simulink model "powertrain"  (R2020b)
settings: Solver=FixedStepAuto  StartTime=0.0  StopTime=t(end)  RelTol=1e-3
PreLoadFcn:
  | C_sc = 1;
StartFcn:
  | C_sc = 1;
values from neighbouring files (symbols this model uses):
  D = 0    [model_fc.m]
  Ts = old_data.Ts    [model_fc.m]
undefined symbols (not defined in the file or in its folder): ANFIS, command, DiscIntNeverNeededParam, ECMS, Flight, in, Ion, Lithium, MPC, out, Tmpc, w
libraries: powerlib x25, neural x25, fuzblock x5, electricdrivelib x3, lib_converters x3, simulink x3, re_lib x1
(part 2 of 8)

== system powertrain/Load1/Flight-1 ==
  In1 : Inport
  1-D Lookup Table1 : Lookup_n-D  NumberOfTableDimensions=1  BreakpointsForDimension1=Break1  Table=Scheme1  InternalRulePriority=Speed  RndMeth=Simplest  InputSameDT=on
  Out1 : Outport
  wires:
  1-D Lookup Table1/1 -> Out1/1
  In1/1 -> 1-D Lookup Table1/1

== system powertrain/Load1/Flight-2 ==
  In1 : Inport
  1-D Lookup Table1 : Lookup_n-D  NumberOfTableDimensions=1  BreakpointsForDimension1=Break2  Table=Scheme2  InternalRulePriority=Speed  RndMeth=Simplest  InputSameDT=on
  Out1 : Outport
  wires:
  1-D Lookup Table1/1 -> Out1/1
  In1/1 -> 1-D Lookup Table1/1

== system powertrain/Load1/Flight-3 ==
  In1 : Inport
  1-D Lookup Table1 : Lookup_n-D  NumberOfTableDimensions=1  BreakpointsForDimension1=Break3  Table=Scheme3  InternalRulePriority=Speed  RndMeth=Simplest  InputSameDT=on
  Out1 : Outport
  wires:
  In1/1 -> 1-D Lookup Table1/1
  1-D Lookup Table1/1 -> Out1/1

== system powertrain/Load1/Flight-noise ==
  In1 : Inport
  1-D Lookup Table1 : Lookup_n-D  NumberOfTableDimensions=1  BreakpointsForDimension1=Break4  Table=Scheme4  InternalRulePriority=Speed  RndMeth=Simplest  InputSameDT=on
  Out1 : Outport
  wires:
  In1/1 -> 1-D Lookup Table1/1
  1-D Lookup Table1/1 -> Out1/1

== system powertrain/Load1/Flight-real ==
  In1 : Inport
  1-D Lookup Table1 : Lookup_n-D  NumberOfTableDimensions=1  BreakpointsForDimension1=Break5  Table=Scheme5  InternalRulePriority=Speed  RndMeth=Simplest  InputSameDT=on
  Out1 : Outport
  wires:
  1-D Lookup Table1/1 -> Out1/1
  In1/1 -> 1-D Lookup Table1/1

== system powertrain/Load1/Step ==
  In1 : Inport
  Step : Step  Time=StepTime  Before=InitVal  After=EndVal
  Out1 : Outport
  wires:
  Step/1 -> Out1/1

== system powertrain/Subsystem/Constant ==
  Constant : Constant  Value=irradiance_const
  Out1 : Outport
  wires:
  Constant/1 -> Out1/1

== system powertrain/Subsystem/Model1 ==
  In1 : Inport
  1-D Lookup Table1 : Lookup_n-D  NumberOfTableDimensions=1  BreakpointsForDimension1=break1  Table=irradiance1  InternalRulePriority=Speed  RndMeth=Simplest  InputSameDT=on
  Out1 : Outport
  wires:
  1-D Lookup Table1/1 -> Out1/1
  In1/1 -> 1-D Lookup Table1/1

== system powertrain/Subsystem/Step ==
  Step : Step  Time=break_step  Before=irradiance_step_init  After=irradiance_step_end  SampleTime=0
  Out1 : Outport
  wires:
  Step/1 -> Out1/1

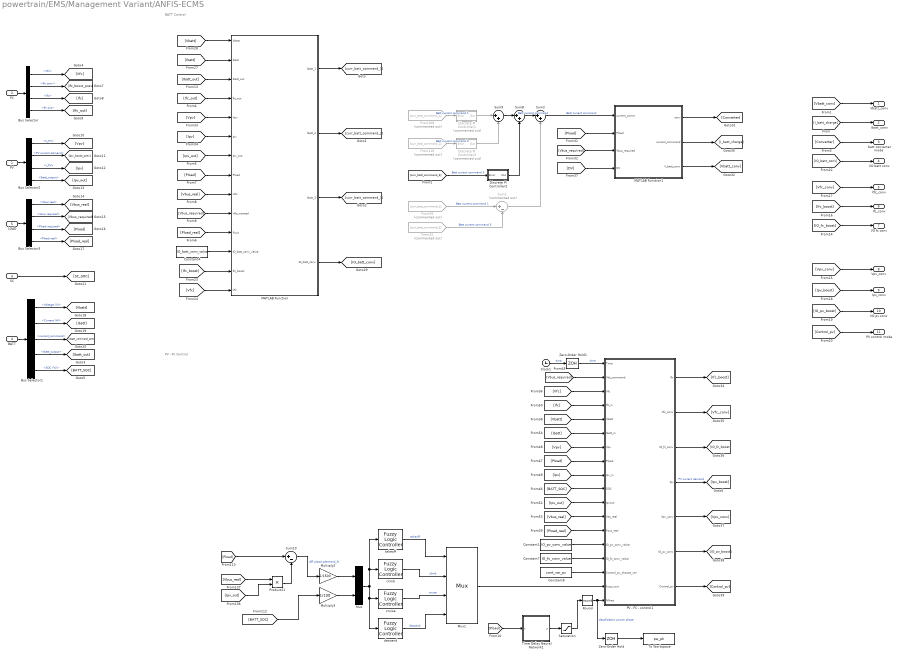
== system powertrain/EMS/Management Variant/ANFIS-ECMS ==
  note: BATT Control
  note: PV - FC Control
  PV : Inport
  FC : Inport  Port=2
  SC : Inport  Port=3
  BATT : Inport  Port=4
  LOAD : Inport  Port=5
  Bus Selector : BusSelector  OutputSignals=Vfc,Ifc conv,Ifc,Ifc out
  Bus Selector1 : BusSelector  OutputSignals=Voltage (V),Current (A),current_command,Ibatt_output,SOC (%)
  Bus Selector2 : BusSelector  OutputSignals=V_PV,PV current demand,I_PV,Ibatt_output
  Bus Selector3 : BusSelector  OutputSignals=Vbus real,Vbus required,Pload required,Pload real
  Clock1 : Clock
  Constant1 : Constant  Value=IO_pv_conv_value
  Constant4 : Constant  Value=IO_batt_conv_value
  Constant7 : Constant  Value=IO_fc_conv_value
  Constant8 : Constant  Value=cont_var_pv
  Discrete PI Controller1 : Subsystem  Commented=on  DialogController=POWERSYS.PowerSysDialog  mask(Discrete PI Controller){Kp=1, Ki=10, Par_Limits=[100 -100], Init=0, Ts=1e-4}
      mask prompts: Kp "Proportional gain (Kp):"; Ki "Integral gain (Ki):"; Par_Limits "Output limits: [ Upper   Lower ]"; Init "Output initial value:"; Ts "Sample time:"
      mask help: This block implements a discrete PI controller.
      mask init:
      | UpperLimit=Par_Limits(1);
      | LowerLimit=Par_Limits(2);
      | power_initmask();
      mask Help: This block is part of a subset of blocks in the Extras library that does not have documentation associated with it, other than the block mask description.
      mask Display: disp('PI');
  Discrete PI Controller2 : Subsystem  DialogController=POWERSYS.PowerSysDialog  mask(Discrete PI Controller){Kp=10, Ki=100, Par_Limits=[30 -4], Init=0, Ts=Ts}
      mask prompts: Kp "Proportional gain (Kp):"; Ki "Integral gain (Ki):"; Par_Limits "Output limits: [ Upper   Lower ]"; Init "Output initial value:"; Ts "Sample time:"
      mask help: This block implements a discrete PI controller.
      mask init:
      | UpperLimit=Par_Limits(1);
      | LowerLimit=Par_Limits(2);
      | power_initmask();
      mask Help: This block is part of a subset of blocks in the Extras library that does not have documentation associated with it, other than the block mask description.
      mask Display: disp('PI');
  Discrete PI Controller3 : Subsystem  Commented=on  DialogController=POWERSYS.PowerSysDialog  mask(Discrete PI Controller){Kp=10, Ki=1, Par_Limits=[100 -100], Init=0, Ts=1e-4}
      mask prompts: Kp "Proportional gain (Kp):"; Ki "Integral gain (Ki):"; Par_Limits "Output limits: [ Upper   Lower ]"; Init "Output initial value:"; Ts "Sample time:"
      mask help: This block implements a discrete PI controller.
      mask init:
      | UpperLimit=Par_Limits(1);
      | LowerLimit=Par_Limits(2);
      | power_initmask();
      mask Help: This block is part of a subset of blocks in the Extras library that does not have documentation associated with it, other than the block mask description.
      mask Display: disp('PI');
  From108 : From  Commented=on  GotoTag=curr_batt_command_1
  From110 : From  Commented=on  GotoTag=curr_batt_command_2
  From25 : From  Commented=on  GotoTag=curr_batt_command_3
  From26 : From  Commented=on  GotoTag=curr_batt_command_1
  MATLAB Function : MATLAB Function  TreatAsAtomicUnit=on
  MATLAB Function1 : MATLAB Function  TreatAsAtomicUnit=on
  Multiply2 : Gain  Gain=1/1500
  Multiply3 : Gain  Gain=1/100
  Mux : Mux  Inputs=2
  Mux1 : Mux
      settings: DisplayOption=signals
  PV - FC - control1 : MATLAB Function  TreatAsAtomicUnit=on
  Product21 : Product
  Round : Rounding  Operator=round
  Saturation : Saturate  UpperLimit=4  LowerLimit=1
  Sum1 : Sum  Commented=on  Inputs=|+-
  Sum10 : Sum  Inputs=|+-
  Sum2 : Sum  Inputs=|++
  Sum8 : Sum  Inputs=|++
  Sum9 : Sum  Inputs=|++
  Time Delay Neural Network1 : Subsystem  mask{pi_input_1_delayed_1=0, pi_input_1_delayed_2=0, pi_input_1_delayed_3=0, pi_input_1_delayed_4=0, pi_input_1_delayed_5=0, pi_input_1_delayed_6=0, pi_input_1_delayed_7=0, pi_input_1_delayed_8=0, pi_input_1_delayed_9=0, pi_input_1_delayed_10=0, pi_input_1_delayed_11=0, pi_input_1_delayed_12=0, pi_input_1_delayed_13=0, pi_input_1_delayed_14=0, pi_input_1_delayed_15=0, pi_input_1_delayed_16=0, pi_input_1_delayed_17=0, pi_input_1_delayed_18=0, pi_input_1_delayed_19=0, pi_input_1_delayed_20=0}
      mask prompts: pi_input_1_delayed_1 "Preprocessed initial input 1 state at timestep 0."; pi_input_1_delayed_2 "Preprocessed initial input 1 state at timestep -1."; pi_input_1_delayed_3 "Preprocessed initial input 1 state at timestep -2."; pi_input_1_delayed_4 "Preprocessed initial input 1 state at timestep -3."; pi_input_1_delayed_5 "Preprocessed initial input 1 state at timestep -4."; pi_input_1_delayed_6 "Preprocessed initial input 1 state at timestep -5."; pi_input_1_delayed_7 "Preprocessed initial input 1 state at timestep -6."; pi_input_1_delayed_8 "Preprocessed initial input 1 state at timestep -7."; pi_input_1_delayed_9 "Preprocessed initial input 1 state at timestep -8."; pi_input_1_delayed_10 "Preprocessed initial input 1 state at timestep -9."; pi_input_1_delayed_11 "Preprocessed initial input 1 state at timestep -10."; pi_input_1_delayed_12 "Preprocessed initial input 1 state at timestep -11."; pi_input_1_delayed_13 "Preprocessed initial input 1 state at timestep -12."; pi_input_1_delayed_14 "Preprocessed initial input 1 state at timestep -13."; pi_input_1_delayed_15 "Preprocessed initial input 1 state at timestep -14."; pi_input_1_delayed_16 "Preprocessed initial input 1 state at timestep -15."; pi_input_1_delayed_17 "Preprocessed initial input 1 state at timestep -16."; pi_input_1_delayed_18 "Preprocessed initial input 1 state at timestep -17."; pi_input_1_delayed_19 "Preprocessed initial input 1 state at timestep -18."; pi_input_1_delayed_20 "Preprocessed initial input 1 state at timestep -19."
      mask help: Time Delay Neural Network
      mask Display: e = 0.06;c1 = [120 150 230]/255;c2 = ([120 150 230]+0)/383;c3 = ([120 150 230]+128)/383;patch([0 1 1 0],[0 0 1 1],c1);patch([0 1 1 1-e 1-e 0+e],[0 0 1 1-e 0+e 0+e],c2);patch([0 0 1 1-e 0+e 0+e],[0 1 1 1-e 1-e 0+e],c3);plot([0 1 1 0 0],[0 0 1 1 0]);fprintf('NNET');port_label('input',1,' x');port_label('output',1,'y ');
  To Workspace : ToWorkspace  VariableName=pw_ph  SaveFormat=Timeseries  SampleTime=-1
  Zero-Order Hold : ZeroOrderHold  SampleTime=Ts
  Zero-Order Hold1 : ZeroOrderHold  SampleTime=Ts
  climb : fuzblock/Fuzzy Logic  Controller  FIS='B80_ECMS_climb.fis'  OutputSampleNumber=10  DataType=double  FuzzifiedInputs=off  RuleFiringStrengths=off  RuleOutputs=off  AggregatedOutputs=off  SimulateUsing=Code generation  OutOfRangeInputValueMessage=warning  NoRuleFiredMessage=warning  EmptyOutputFuzzySetMessage=warning
  cruise : fuzblock/Fuzzy Logic  Controller  FIS='B80_ECMS_cruise.fis'  OutputSampleNumber=10  DataType=double  FuzzifiedInputs=off  RuleFiringStrengths=off  RuleOutputs=off  AggregatedOutputs=off  SimulateUsing=Code generation  OutOfRangeInputValueMessage=warning  NoRuleFiredMessage=warning  EmptyOutputFuzzySetMessage=warning
  descend : fuzblock/Fuzzy Logic  Controller  FIS='B80_ECMS_descend.fis'  OutputSampleNumber=10  DataType=double  FuzzifiedInputs=off  RuleFiringStrengths=off  RuleOutputs=off  AggregatedOutputs=off  SimulateUsing=Code generation  OutOfRangeInputValueMessage=warning  NoRuleFiredMessage=warning  EmptyOutputFuzzySetMessage=warning
  takeoff : fuzblock/Fuzzy Logic  Controller  FIS='B80_ECMS_takeoff.fis'  OutputSampleNumber=10  DataType=double  FuzzifiedInputs=off  RuleFiringStrengths=off  RuleOutputs=off  AggregatedOutputs=off  SimulateUsing=Code generation  OutOfRangeInputValueMessage=warning  NoRuleFiredMessage=warning  EmptyOutputFuzzySetMessage=warning
  Vbatt_conv : Outport
  Ibatt_conv : Outport  Port=2
  batt converter mode : Outport  Port=3
  I/O batt conv : Outport  Port=4
  Vfc_conv : Outport  Port=5
  Ifc_conv : Outport  Port=6
  I/O fc conv : Outport  Port=7
  Vpv_conv : Outport  Port=8
  Ipv_conv : Outport  Port=9
  I/O pv conv : Outport  Port=10
  PV control mode : Outport  Port=11
  wires:
  [DV] -> MATLAB Function1/4(DV)
  Discrete PI Controller1/1(Out) -> Sum9/1
  [I_batt_charge] -> Ibatt_conv/1
  MATLAB Function1/1(conv) -> [Converter]
  [Converter] -> batt converter mode/1
  Sum9/1 -> Sum8/1
  Bus Selector1/1 -> [Vbatt]  "<Voltage (V)>"
  [Vbus_real] -> MATLAB Function/9(Vdc)
  [Vpv] -> MATLAB Function/5(Vpv)
  Bus Selector/1 -> [Vfc]  "<Vfc>"
  Sum2/1 -> MATLAB Function1/1(current_comm)  "Batt current command"
  [Vfc_conv] -> Vfc_conv/1
  BATT/1 -> Bus Selector1/1
  From25/1 -> Sum1/2  "Batt current command 3"
  MATLAB Function/3(Ibatt_3) -> [curr_batt_command_3]
  [Vfc] -> MATLAB Function/14(Vfc)
  Bus Selector2/3 -> [Ipv]  "<I_PV>"
  [IO_pv_boost] -> I/O pv conv/1
  From108/1 -> Discrete PI Controller1/1(Error)  "Batt current command 1"
  [Ibatt] -> MATLAB Function/2(Ibatt)
  [IO_fc_boost] -> I/O fc conv/1
  MATLAB Function/2(Ibatt_2) -> [curr_batt_command_2]
  Constant4/1 -> MATLAB Function/12(IO_batt_conv_value)
  MATLAB Function/1(Ibatt_1) -> [curr_batt_command_1]
  [Pload] -> MATLAB Function1/2(Pload)
  Bus Selector2/1 -> [Vpv]  "<V_PV>"
  [Ipv] -> MATLAB Function/6(Ipv)
  SC/1 -> [SC_SOC]
  [Ibatt_out] -> MATLAB Function/3(Ibatt_out)
  MATLAB Function1/2(current_command) -> [I_batt_charge]
  [Pload_real] -> MATLAB Function/11(Pout)
  From26/1 -> Sum1/1  "Batt current command 1"
  Bus Selector/4 -> [Ifc_out]  "<Ifc out>"
  FC/1 -> Bus Selector/1
  Bus Selector2/2 -> [Ipv_boost_prev]  "<PV current demand>"
  Bus Selector3/1 -> [Vbus_real]  "<Vbus real>"
  Bus Selector3/2 -> [Vbus_required]  "<Vbus required>"
  [Ipv_boost] -> Ipv_conv/1
  Bus Selector1/4 -> [Ibatt_out]  "<Ibatt_output>"
  Bus Selector1/5 -> [BATT_SOC]  "<SOC (%)>"
  Discrete PI Controller2/1(Out) -> Sum8/2
  [Vbatt] -> MATLAB Function/1(Vbatt)
  Discrete PI Controller3/1(Out) -> Sum9/2
  Bus Selector3/4 -> [Pload_real]  "<Pload real>"
  Bus Selector/2 -> [Ifc_boost_prev]  "<Ifc conv>"
  [Ifc_boost] -> MATLAB Function/13(Ifc_boost)
  MATLAB Function1/3(V_batt_conv) -> [Vbatt_conv]
  Bus Selector1/2 -> [Ibatt]  "<Current (A)>"
  [Vpv_conv] -> Vpv_conv/1
  [Ifc_out] -> MATLAB Function/4(Ifc_out)
  Bus Selector1/3 -> [Ibatt_command_pre]  "<current_command>"
  [Vbus_required] -> MATLAB Function1/3(Vbus_required)
  From110/1 -> Discrete PI Controller3/1(Error)  "Batt current command 3"
  [curr_batt_command_3] -> Discrete PI Controller2/1(Error)  "Batt current command 3"
  PV/1 -> Bus Selector2/1
  [Vbus_required] -> MATLAB Function/10(Vdc_wanted)
  Bus Selector2/4 -> [Ipv_out]  "<Ibatt_output>"
  Bus Selector3/3 -> [Pload]  "<Pload required>"
  [IO_batt_conv] -> I/O batt conv/1
  Bus Selector/3 -> [Ifc]  "<Ifc>"
  [Ipv_out] -> MATLAB Function/7(Ipv_out)
  [Control_pv] -> PV control mode/1
  LOAD/1 -> Bus Selector3/1
  Sum8/1 -> Sum2/1  "Batt current command"
  [Pload] -> MATLAB Function/8(Pload)
  [Vbatt_conv] -> Vbatt_conv/1
  MATLAB Function/4(IO_batt_conv) -> [IO_batt_conv]
  Sum1/1 -> Sum2/2
  [Vbus_real] -> Product21/1
  takeoff/1 -> Mux1/1  "takeoff"
  [BATT_SOC] -> Multiply3/1
  Multiply2/1 -> Mux/1
  [Pload] -> Sum10/1
  Product21/1 -> Sum10/2
  Mux/1 -> takeoff/1, climb/1, descend/1, cruise/1
  Sum10/1 -> Multiply2/1  "diff pload pdemand_fc"
  [Ipv_out] -> Product21/2
  Multiply3/1 -> Mux/2
  Mux1/1 -> PV - FC - control1/17(fuzzy_out)
  PV - FC - control1/1(Ifc) -> [Ifc_boost]
  Zero-Order Hold1/1 -> PV - FC - control1/1(Time)  "time"
  [Pload] -> PV - FC - control1/8(Pload)
  Constant7/1 -> PV - FC - control1/15(IO_fc_conv_value)
  [BATT_SOC] -> PV - FC - control1/10(SOC)
  [Vbatt] -> PV - FC - control1/5(Vbatt)
  [Ibatt] -> PV - FC - control1/6(Ibatt_in)
  PV - FC - control1/5(Vpv_conv) -> [Vpv_conv]
  PV - FC - control1/2(Vfc_conv) -> [Vfc_conv]
  [Vfc] -> PV - FC - control1/3(Vfc)
  PV - FC - control1/4(Ipv) -> [Ipv_boost]  "PV current demand"
  [Ifc] -> PV - FC - control1/4(Ifc_in)
  Constant8/1 -> PV - FC - control1/16(Control_pv_choose_var)
  [Ipv] -> PV - FC - control1/9(Ipv_in)
  PV - FC - control1/6(IO_pv_conv) -> [IO_pv_boost]
  [Pload_real] -> PV - FC - control1/13(Pout_real)
  PV - FC - control1/7(Control_pv) -> [Control_pv]
  [Vbus_real] -> PV - FC - control1/12(Vdc_real)
  [Vpv] -> PV - FC - control1/7(Vpv)
  Constant1/1 -> PV - FC - control1/14(IO_pv_conv_value)
  [Ipv_out] -> PV - FC - control1/11(Ipvout)
  Clock1/1 -> Zero-Order Hold1/1  "time"
  [Vbus_required] -> PV - FC - control1/2(Vdc_command)
  PV - FC - control1/3(IO_fc_conv) -> [IO_fc_boost]
  climb/1 -> Mux1/2  "climb"
  cruise/1 -> Mux1/3  "cruise"
  descend/1 -> Mux1/4  "descend"
  Time Delay Neural Network1/1(y) -> Saturation/1
  [Pload] -> Time Delay Neural Network1/1(x)
  Saturation/1 -> Round/1
  Round/1 -> Zero-Order Hold/1, PV - FC - control1/18(NNres)  "classficiation power phase"
  [Ifc_boost] -> Ifc_conv/1
  Zero-Order Hold/1 -> To Workspace/1

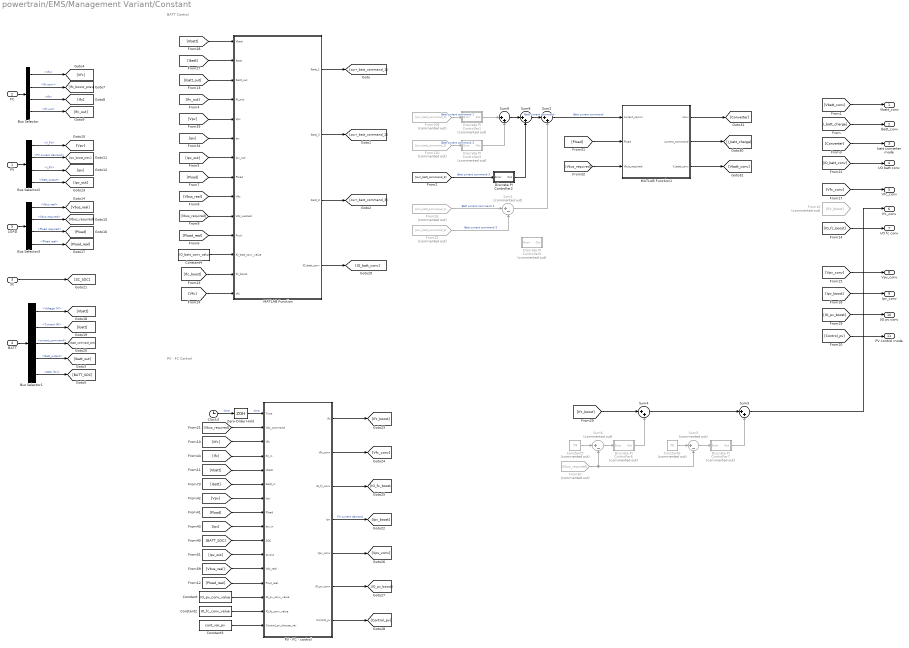
== system powertrain/EMS/Management Variant/Constant ==
  note: BATT Control
  note: PV - FC Control
  PV : Inport
  FC : Inport  Port=2
  SC : Inport  Port=3
  BATT : Inport  Port=4
  LOAD : Inport  Port=5
  Bus Selector : BusSelector  OutputSignals=Vfc,Ifc conv,Ifc,Ifc out
  Bus Selector1 : BusSelector  OutputSignals=Voltage (V),Current (A),current_command,Ibatt_output,SOC (%)
  Bus Selector2 : BusSelector  OutputSignals=V_PV,PV current demand,I_PV,Ibatt_output
  Bus Selector3 : BusSelector  OutputSignals=Vbus real,Vbus required,Pload required,Pload real
  Clock3 : Clock
  Constant : Constant  Value=IO_pv_conv_value
  Constant2 : Constant  Value=IO_fc_conv_value
  Constant3 : Constant  Value=cont_var_pv
  Constant4 : Constant  Value=IO_batt_conv_value
  Constant5 : Constant  Commented=on  Value=74
  Constant6 : Constant  Commented=on  Value=70
  Discrete PI Controller1 : Subsystem  Commented=on  DialogController=POWERSYS.PowerSysDialog  mask(Discrete PI Controller){Kp=1, Ki=10, Par_Limits=[100 -100], Init=0, Ts=1e-4}
      mask prompts: Kp "Proportional gain (Kp):"; Ki "Integral gain (Ki):"; Par_Limits "Output limits: [ Upper   Lower ]"; Init "Output initial value:"; Ts "Sample time:"
      mask help: This block implements a discrete PI controller.
      mask init:
      | UpperLimit=Par_Limits(1);
      | LowerLimit=Par_Limits(2);
      | power_initmask();
      mask Help: This block is part of a subset of blocks in the Extras library that does not have documentation associated with it, other than the block mask description.
      mask Display: disp('PI');
  Discrete PI Controller2 : Subsystem  DialogController=POWERSYS.PowerSysDialog  mask(Discrete PI Controller){Kp=10, Ki=100, Par_Limits=[30 -4], Init=0, Ts=Ts}
      mask prompts: Kp "Proportional gain (Kp):"; Ki "Integral gain (Ki):"; Par_Limits "Output limits: [ Upper   Lower ]"; Init "Output initial value:"; Ts "Sample time:"
      mask help: This block implements a discrete PI controller.
      mask init:
      | UpperLimit=Par_Limits(1);
      | LowerLimit=Par_Limits(2);
      | power_initmask();
      mask Help: This block is part of a subset of blocks in the Extras library that does not have documentation associated with it, other than the block mask description.
      mask Display: disp('PI');
  Discrete PI Controller3 : Subsystem  Commented=on  DialogController=POWERSYS.PowerSysDialog  mask(Discrete PI Controller){Kp=10, Ki=1, Par_Limits=[100 -100], Init=0, Ts=1e-4}
      mask prompts: Kp "Proportional gain (Kp):"; Ki "Integral gain (Ki):"; Par_Limits "Output limits: [ Upper   Lower ]"; Init "Output initial value:"; Ts "Sample time:"
      mask help: This block implements a discrete PI controller.
      mask init:
      | UpperLimit=Par_Limits(1);
      | LowerLimit=Par_Limits(2);
      | power_initmask();
      mask Help: This block is part of a subset of blocks in the Extras library that does not have documentation associated with it, other than the block mask description.
      mask Display: disp('PI');
  Discrete PI Controller5 : Subsystem  Commented=on  DialogController=POWERSYS.PowerSysDialog  mask(Discrete PI Controller){Kp=10, Ki=10, Par_Limits=[50 -20], Init=0, Ts=1e-4}
      mask prompts: Kp "Proportional gain (Kp):"; Ki "Integral gain (Ki):"; Par_Limits "Output limits: [ Upper   Lower ]"; Init "Output initial value:"; Ts "Sample time:"
      mask help: This block implements a discrete PI controller.
      mask init:
      | UpperLimit=Par_Limits(1);
      | LowerLimit=Par_Limits(2);
      | power_initmask();
      mask Help: This block is part of a subset of blocks in the Extras library that does not have documentation associated with it, other than the block mask description.
      mask Display: disp('PI');
  Discrete PI Controller6 : Subsystem  Commented=on  DialogController=POWERSYS.PowerSysDialog  mask(Discrete PI Controller){Kp=10, Ki=10, Par_Limits=[40 0], Init=0, Ts=1e-4}
      mask prompts: Kp "Proportional gain (Kp):"; Ki "Integral gain (Ki):"; Par_Limits "Output limits: [ Upper   Lower ]"; Init "Output initial value:"; Ts "Sample time:"
      mask help: This block implements a discrete PI controller.
      mask init:
      | UpperLimit=Par_Limits(1);
      | LowerLimit=Par_Limits(2);
      | power_initmask();
      mask Help: This block is part of a subset of blocks in the Extras library that does not have documentation associated with it, other than the block mask description.
      mask Display: disp('PI');
  Discrete PI Controller7 : Subsystem  Commented=on  DialogController=POWERSYS.PowerSysDialog  mask(Discrete PI Controller){Kp=10, Ki=10, Par_Limits=[0 -40], Init=0, Ts=1e-4}
      mask prompts: Kp "Proportional gain (Kp):"; Ki "Integral gain (Ki):"; Par_Limits "Output limits: [ Upper   Lower ]"; Init "Output initial value:"; Ts "Sample time:"
      mask help: This block implements a discrete PI controller.
      mask init:
      | UpperLimit=Par_Limits(1);
      | LowerLimit=Par_Limits(2);
      | power_initmask();
      mask Help: This block is part of a subset of blocks in the Extras library that does not have documentation associated with it, other than the block mask description.
      mask Display: disp('PI');
  From108 : From  Commented=on  GotoTag=curr_batt_command_1
  From110 : From  Commented=on  GotoTag=curr_batt_command_2
  From16 : From  Commented=on  GotoTag=Ifc_boost
  From25 : From  Commented=on  GotoTag=curr_batt_command_3
  From26 : From  Commented=on  GotoTag=curr_batt_command_1
  From30 : From  Commented=on  GotoTag=Vbus_required
  MATLAB Function : MATLAB Function  TreatAsAtomicUnit=on
  MATLAB Function1 : MATLAB Function  TreatAsAtomicUnit=on
  PV - FC - control : MATLAB Function  TreatAsAtomicUnit=on
  Sum1 : Sum  Commented=on  Inputs=|+-
  Sum{2..4,8..9} (5 alike) : Sum  Inputs=|++
  Sum5 : Sum  Commented=on  Inputs=|+-
  Sum6 : Sum  Commented=on  Inputs=|+-
  Zero-Order Hold : ZeroOrderHold  SampleTime=1e-4
  Vbatt_conv : Outport
  Ibatt_conv : Outport  Port=2
  batt converter mode : Outport  Port=3
  I/O batt conv : Outport  Port=4
  Vfc_conv : Outport  Port=5
  Ifc_conv : Outport  Port=6
  I/O fc conv : Outport  Port=7
  Vpv_conv : Outport  Port=8
  Ipv_conv : Outport  Port=9
  I/O pv conv : Outport  Port=10
  PV control mode : Outport  Port=11
  wires:
  Constant/1 -> PV - FC - control/14(IO_pv_conv_value)
  MATLAB Function1/1(conv) -> [Converter]
  [Vbatt] -> MATLAB Function/1(Vbatt)
  [Ibatt_out] -> MATLAB Function/3(Ibatt_out)
  Bus Selector1/5 -> [BATT_SOC]  "<SOC (%)>"
  From30/1 -> Sum5/2, Sum6/2
  [Vpv] -> MATLAB Function/5(Vpv)
  Sum6/1 -> Discrete PI Controller6/1(Error)
  Discrete PI Controller7/1(Out) -> Sum3/2
  PV - FC - control/3(IO_fc_conv) -> [IO_fc_boost]
  [Ifc_out] -> MATLAB Function/4(Ifc_out)
  Bus Selector1/3 -> [Ibatt_command_pre]  "<current_command>"
  [IO_fc_boost] -> I/O fc conv/1
  MATLAB Function1/3(V_batt_conv) -> [Vbatt_conv]
  Bus Selector1/2 -> [Ibatt]  "<Current (A)>"
  [Ifc_boost] -> MATLAB Function/13(Ifc_boost)
  [Vbus_required] -> MATLAB Function1/3(Vbus_required)
  Sum2/1 -> MATLAB Function1/1(current_comm)  "Batt current command"
  [Vpv_conv] -> Vpv_conv/1
  Bus Selector1/1 -> [Vbatt]  "<Voltage (V)>"
  [Ibatt] -> PV - FC - control/6(Ibatt_in)
  From26/1 -> Sum1/1  "Batt current command 1"
  Bus Selector1/4 -> [Ibatt_out]  "<Ibatt_output>"
  MATLAB Function1/2(current_command) -> [I_batt_charge]
  [Ipv_boost] -> Ipv_conv/1
  [Pload_real] -> MATLAB Function/11(Pout)
  PV - FC - control/5(Vpv_conv) -> [Vpv_conv]
  Constant6/1 -> Sum5/1
  Sum5/1 -> Discrete PI Controller7/1(Error)
  Constant2/1 -> PV - FC - control/15(IO_fc_conv_value)
  MATLAB Function/2(Ibatt_2) -> [curr_batt_command_2]
  MATLAB Function/1(Ibatt_1) -> [curr_batt_command_1]
  Bus Selector2/1 -> [Vpv]  "<V_PV>"
  [Pload] -> MATLAB Function1/2(Pload)
  Sum4/1 -> Sum3/1
  [Ifc_boost] -> Sum4/1
  From25/1 -> Sum1/2  "Batt current command 3"
  [Ibatt] -> MATLAB Function/2(Ibatt)
  [IO_pv_boost] -> I/O pv conv/1
  [Vfc] -> MATLAB Function/14(Vfc)
  Bus Selector2/3 -> [Ipv]  "<I_PV>"
  Sum1/1 -> Sum2/2
  [Vfc_conv] -> Vfc_conv/1
  [Ipv_out] -> PV - FC - control/11(Ipvout)
  PV - FC - control/7(Control_pv) -> [Control_pv]
  [Vbus_required] -> PV - FC - control/2(Vdc_command)
  [Vbatt_conv] -> Vbatt_conv/1
  [Vbus_real] -> PV - FC - control/12(Vdc_real)
  MATLAB Function/4(IO_batt_conv) -> [IO_batt_conv]
  Constant3/1 -> PV - FC - control/16(Control_pv_choose_var)
  PV - FC - control/1(Ifc) -> [Ifc_boost]
  FC/1 -> Bus Selector/1
  [Ipv] -> PV - FC - control/9(Ipv_in)
  Sum8/1 -> Sum2/1  "Batt current command"
  Zero-Order Hold/1 -> PV - FC - control/1(Time)  "time"
  [Pload] -> MATLAB Function/8(Pload)
  [Vbus_required] -> MATLAB Function/10(Vdc_wanted)
  Clock3/1 -> Zero-Order Hold/1  "time"
  [Pload_real] -> PV - FC - control/13(Pout_real)
  [Vpv] -> PV - FC - control/7(Vpv)
  LOAD/1 -> Bus Selector3/1
  Constant5/1 -> Sum6/1
  [Control_pv] -> PV control mode/1
  Bus Selector/3 -> [Ifc]  "<Ifc>"
  [Ipv_out] -> MATLAB Function/7(Ipv_out)
  From110/1 -> Discrete PI Controller3/1(Error)  "Batt current command 3"
  [IO_batt_conv] -> I/O batt conv/1
  [Vbus_real] -> MATLAB Function/9(Vdc)
  Bus Selector3/3 -> [Pload]  "<Pload required>"
  Bus Selector2/4 -> [Ipv_out]  "<Ibatt_output>"
  PV - FC - control/4(Ipv) -> [Ipv_boost]  "PV current demand"
  [Ifc] -> PV - FC - control/4(Ifc_in)
  Bus Selector3/2 -> [Vbus_required]  "<Vbus required>"
  BATT/1 -> Bus Selector1/1
  Discrete PI Controller6/1(Out) -> Sum4/2
  Bus Selector2/2 -> [Ipv_boost_prev]  "<PV current demand>"
  Bus Selector3/1 -> [Vbus_real]  "<Vbus real>"
  Constant4/1 -> MATLAB Function/12(IO_batt_conv_value)
  PV - FC - control/6(IO_pv_conv) -> [IO_pv_boost]
  SC/1 -> [SC_SOC]
  [Converter] -> batt converter mode/1
  PV - FC - control/2(Vfc_conv) -> [Vfc_conv]
  [I_batt_charge] -> Ibatt_conv/1
  [Vbatt] -> PV - FC - control/5(Vbatt)
  [Vfc] -> PV - FC - control/3(Vfc)
  [curr_batt_command_3] -> Discrete PI Controller2/1(Error)  "Batt current command 3"
  Bus Selector/1 -> [Vfc]  "<Vfc>"
  Bus Selector/4 -> [Ifc_out]  "<Ifc out>"
  PV/1 -> Bus Selector2/1
  [Pload] -> PV - FC - control/8(Pload)
  Bus Selector/2 -> [Ifc_boost_prev]  "<Ifc conv>"
  Sum9/1 -> Sum8/1
  From108/1 -> Discrete PI Controller1/1(Error)  "Batt current command 1"
  Discrete PI Controller2/1(Out) -> Sum8/2
  MATLAB Function/3(Ibatt_3) -> [curr_batt_command_3]
  Sum3/1 -> Ifc_conv/1
  Discrete PI Controller1/1(Out) -> Sum9/1
  Discrete PI Controller3/1(Out) -> Sum9/2
  [BATT_SOC] -> PV - FC - control/10(SOC)
  [Ipv] -> MATLAB Function/6(Ipv)
  Bus Selector3/4 -> [Pload_real]  "<Pload real>"

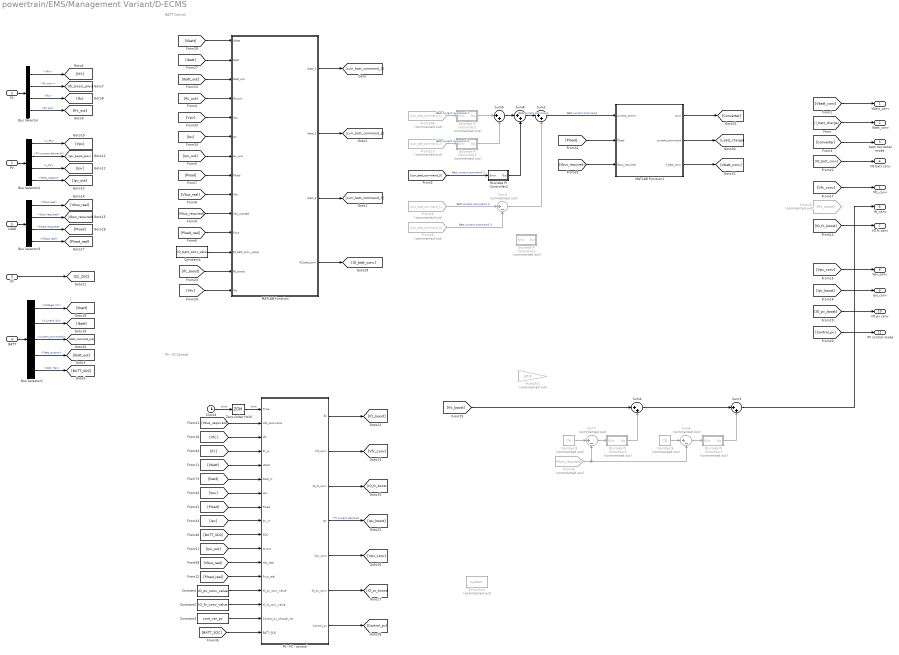
== system powertrain/EMS/Management Variant/D-ECMS ==
  note: PV - FC Control
  note: BATT Control
  PV : Inport
  FC : Inport  Port=2
  SC : Inport  Port=3
  BATT : Inport  Port=4
  LOAD : Inport  Port=5
  Bus Selector : BusSelector  OutputSignals=Vfc,Ifc conv,Ifc,Ifc out
  Bus Selector1 : BusSelector  OutputSignals=Voltage (V),Current (A),current_command,Ibatt_output,SOC (%)
  Bus Selector2 : BusSelector  OutputSignals=V_PV,PV current demand,I_PV,Ibatt_output
  Bus Selector3 : BusSelector  OutputSignals=Vbus real,Vbus required,Pload required,Pload real
  Clock3 : Clock
  Constant : Constant  Value=IO_pv_conv_value
  Constant2 : Constant  Value=IO_fc_conv_value
  Constant3 : Constant  Value=cont_var_pv
  Constant4 : Constant  Value=IO_batt_conv_value
  Constant5 : Constant  Commented=on  Value=74
  Constant6 : Constant  Commented=on  Value=70
  Discrete PI Controller1 : Subsystem  Commented=on  DialogController=POWERSYS.PowerSysDialog  mask(Discrete PI Controller){Kp=1, Ki=10, Par_Limits=[100 -100], Init=0, Ts=1e-4}
      mask prompts: Kp "Proportional gain (Kp):"; Ki "Integral gain (Ki):"; Par_Limits "Output limits: [ Upper   Lower ]"; Init "Output initial value:"; Ts "Sample time:"
      mask help: This block implements a discrete PI controller.
      mask init:
      | UpperLimit=Par_Limits(1);
      | LowerLimit=Par_Limits(2);
      | power_initmask();
      mask Help: This block is part of a subset of blocks in the Extras library that does not have documentation associated with it, other than the block mask description.
      mask Display: disp('PI');
  Discrete PI Controller2 : Subsystem  DialogController=POWERSYS.PowerSysDialog  mask(Discrete PI Controller){Kp=10, Ki=100, Par_Limits=[30 -4], Init=0, Ts=Ts}
      mask prompts: Kp "Proportional gain (Kp):"; Ki "Integral gain (Ki):"; Par_Limits "Output limits: [ Upper   Lower ]"; Init "Output initial value:"; Ts "Sample time:"
      mask help: This block implements a discrete PI controller.
      mask init:
      | UpperLimit=Par_Limits(1);
      | LowerLimit=Par_Limits(2);
      | power_initmask();
      mask Help: This block is part of a subset of blocks in the Extras library that does not have documentation associated with it, other than the block mask description.
      mask Display: disp('PI');
  Discrete PI Controller3 : Subsystem  Commented=on  DialogController=POWERSYS.PowerSysDialog  mask(Discrete PI Controller){Kp=10, Ki=1, Par_Limits=[100 -100], Init=0, Ts=1e-4}
      mask prompts: Kp "Proportional gain (Kp):"; Ki "Integral gain (Ki):"; Par_Limits "Output limits: [ Upper   Lower ]"; Init "Output initial value:"; Ts "Sample time:"
      mask help: This block implements a discrete PI controller.
      mask init:
      | UpperLimit=Par_Limits(1);
      | LowerLimit=Par_Limits(2);
      | power_initmask();
      mask Help: This block is part of a subset of blocks in the Extras library that does not have documentation associated with it, other than the block mask description.
      mask Display: disp('PI');
  Discrete PI Controller5 : Subsystem  Commented=on  DialogController=POWERSYS.PowerSysDialog  mask(Discrete PI Controller){Kp=10, Ki=10, Par_Limits=[50 -20], Init=0, Ts=1e-4}
      mask prompts: Kp "Proportional gain (Kp):"; Ki "Integral gain (Ki):"; Par_Limits "Output limits: [ Upper   Lower ]"; Init "Output initial value:"; Ts "Sample time:"
      mask help: This block implements a discrete PI controller.
      mask init:
      | UpperLimit=Par_Limits(1);
      | LowerLimit=Par_Limits(2);
      | power_initmask();
      mask Help: This block is part of a subset of blocks in the Extras library that does not have documentation associated with it, other than the block mask description.
      mask Display: disp('PI');
  Discrete PI Controller6 : Subsystem  Commented=on  DialogController=POWERSYS.PowerSysDialog  mask(Discrete PI Controller){Kp=10, Ki=10, Par_Limits=[40 0], Init=0, Ts=1e-4}
      mask prompts: Kp "Proportional gain (Kp):"; Ki "Integral gain (Ki):"; Par_Limits "Output limits: [ Upper   Lower ]"; Init "Output initial value:"; Ts "Sample time:"
      mask help: This block implements a discrete PI controller.
      mask init:
      | UpperLimit=Par_Limits(1);
      | LowerLimit=Par_Limits(2);
      | power_initmask();
      mask Help: This block is part of a subset of blocks in the Extras library that does not have documentation associated with it, other than the block mask description.
      mask Display: disp('PI');
  Discrete PI Controller7 : Subsystem  Commented=on  DialogController=POWERSYS.PowerSysDialog  mask(Discrete PI Controller){Kp=10, Ki=10, Par_Limits=[0 -40], Init=0, Ts=1e-4}
      mask prompts: Kp "Proportional gain (Kp):"; Ki "Integral gain (Ki):"; Par_Limits "Output limits: [ Upper   Lower ]"; Init "Output initial value:"; Ts "Sample time:"
      mask help: This block implements a discrete PI controller.
      mask init:
      | UpperLimit=Par_Limits(1);
      | LowerLimit=Par_Limits(2);
      | power_initmask();
      mask Help: This block is part of a subset of blocks in the Extras library that does not have documentation associated with it, other than the block mask description.
      mask Display: disp('PI');
  From108 : From  Commented=on  GotoTag=curr_batt_command_1
  From110 : From  Commented=on  GotoTag=curr_batt_command_2
  From16 : From  Commented=on  GotoTag=Ifc_boost
  From25 : From  Commented=on  GotoTag=curr_batt_command_3
  From26 : From  Commented=on  GotoTag=curr_batt_command_1
  From30 : From  Commented=on  GotoTag=Vbus_required
  MATLAB Function : MATLAB Function  TreatAsAtomicUnit=on
  MATLAB Function1 : MATLAB Function  TreatAsAtomicUnit=on
  Multiply1 : Gain  Commented=on  Gain=1/0.9
  PV - FC - control : MATLAB Function  TreatAsAtomicUnit=on
  S-Function : S-Function  Commented=on  SFunctionDeploymentMode=off  EnableBusSupport=off
  Sum1 : Sum  Commented=on  Inputs=|+-
  Sum{2..4,8..9} (5 alike) : Sum  Inputs=|++
  Sum6 : Sum  Commented=on  Inputs=|+-
  Sum7 : Sum  Commented=on  Inputs=|+-
  Zero-Order Hold : ZeroOrderHold  SampleTime=Ts
  Vbatt_conv : Outport
  Ibatt_conv : Outport  Port=2
  batt converter mode : Outport  Port=3
  I/O batt conv : Outport  Port=4
  Vfc_conv : Outport  Port=5
  Ifc_conv : Outport  Port=6
  I/O fc conv : Outport  Port=7
  Vpv_conv : Outport  Port=8
  Ipv_conv : Outport  Port=9
  I/O pv conv : Outport  Port=10
  PV control mode : Outport  Port=11
  wires:
  [Ipv_out] -> PV - FC - control/11(Ipvout)
  Sum1/1 -> Sum2/2
  PV - FC - control/7(Control_pv) -> [Control_pv]
  [Vbus_required] -> PV - FC - control/2(Vdc_command)
  MATLAB Function/4(IO_batt_conv) -> [IO_batt_conv]
  Constant3/1 -> PV - FC - control/16(Control_pv_choose_var)
  [Vbatt_conv] -> Vbatt_conv/1
  [Vbus_real] -> PV - FC - control/12(Vdc_real)
  [Pload] -> MATLAB Function/8(Pload)
  Zero-Order Hold/1 -> PV - FC - control/1(Time)  "time"
  [Ipv] -> PV - FC - control/9(Ipv_in)
  Sum8/1 -> Sum2/1  "Batt current command"
  [Vpv] -> PV - FC - control/7(Vpv)
  LOAD/1 -> Bus Selector3/1
  Clock3/1 -> Zero-Order Hold/1  "time"
  [Control_pv] -> PV control mode/1
  [Ipv_out] -> MATLAB Function/7(Ipv_out)
  Bus Selector/3 -> [Ifc]  "<Ifc>"
  [IO_batt_conv] -> I/O batt conv/1
  Bus Selector3/3 -> [Pload]  "<Pload required>"
  PV - FC - control/4(Ipv) -> [Ipv_boost]  "PV current demand"
  Bus Selector2/4 -> [Ipv_out]  "<Ibatt_output>"
  [Ifc_boost] -> Sum4/1
  [Vbus_required] -> MATLAB Function/10(Vdc_wanted)
  [BATT_SOC] -> PV - FC - control/17(BATT_SOC)
  PV/1 -> Bus Selector2/1
  [curr_batt_command_3] -> Discrete PI Controller2/1(Error)  "Batt current command 3"
  From110/1 -> Discrete PI Controller3/1(Error)  "Batt current command 3"
  [Vbus_required] -> MATLAB Function1/3(Vbus_required)
  Bus Selector1/3 -> [Ibatt_command_pre]  "<current_command>"
  PV - FC - control/3(IO_fc_conv) -> [IO_fc_boost]
  [Ifc_out] -> MATLAB Function/4(Ifc_out)
  [Vpv_conv] -> Vpv_conv/1
  Bus Selector1/2 -> [Ibatt]  "<Current (A)>"
  MATLAB Function1/3(V_batt_conv) -> [Vbatt_conv]
  [Ifc_boost] -> MATLAB Function/13(Ifc_boost)
  Bus Selector/2 -> [Ifc_boost_prev]  "<Ifc conv>"
  Bus Selector3/4 -> [Pload_real]  "<Pload real>"
  Discrete PI Controller3/1(Out) -> Sum9/2
  [Ifc] -> PV - FC - control/4(Ifc_in)
  Discrete PI Controller6/1(Out) -> Sum4/2
  [Vbatt] -> MATLAB Function/1(Vbatt)
  PV - FC - control/6(IO_pv_conv) -> [IO_pv_boost]
  Discrete PI Controller2/1(Out) -> Sum8/2
  Bus Selector1/5 -> [BATT_SOC]  "<SOC (%)>"
  Bus Selector1/4 -> [Ibatt_out]  "<Ibatt_output>"
  [Vbatt] -> PV - FC - control/5(Vbatt)
  [Ipv_boost] -> Ipv_conv/1
  Sum7/1 -> Discrete PI Controller6/1(Error)
  Bus Selector3/2 -> [Vbus_required]  "<Vbus required>"
  Bus Selector3/1 -> [Vbus_real]  "<Vbus real>"
  Bus Selector2/2 -> [Ipv_boost_prev]  "<PV current demand>"
  FC/1 -> Bus Selector/1
  PV - FC - control/2(Vfc_conv) -> [Vfc_conv]
  Bus Selector/4 -> [Ifc_out]  "<Ifc out>"
  PV - FC - control/1(Ifc) -> [Ifc_boost]
  [BATT_SOC] -> PV - FC - control/10(SOC)
  [Vfc] -> PV - FC - control/3(Vfc)
  [Pload] -> PV - FC - control/8(Pload)
  Sum6/1 -> Discrete PI Controller7/1(Error)
  From26/1 -> Sum1/1  "Batt current command 1"
  [Pload_real] -> MATLAB Function/11(Pout)
  PV - FC - control/5(Vpv_conv) -> [Vpv_conv]
  MATLAB Function1/2(current_command) -> [I_batt_charge]
  [Ibatt_out] -> MATLAB Function/3(Ibatt_out)
  Constant6/1 -> Sum6/1
  Sum4/1 -> Sum3/1
  SC/1 -> [SC_SOC]
  [Ipv] -> MATLAB Function/6(Ipv)
  Bus Selector2/1 -> [Vpv]  "<V_PV>"
  Constant2/1 -> PV - FC - control/15(IO_fc_conv_value)
  [Pload] -> MATLAB Function1/2(Pload)
  MATLAB Function/1(Ibatt_1) -> [curr_batt_command_1]
  Constant5/1 -> Sum7/1
  Constant4/1 -> MATLAB Function/12(IO_batt_conv_value)
  MATLAB Function/2(Ibatt_2) -> [curr_batt_command_2]
  [IO_fc_boost] -> I/O fc conv/1
  [Ibatt] -> MATLAB Function/2(Ibatt)
  From108/1 -> Discrete PI Controller1/1(Error)  "Batt current command 1"
  [IO_pv_boost] -> I/O pv conv/1
  Bus Selector2/3 -> [Ipv]  "<I_PV>"
  [Vfc] -> MATLAB Function/14(Vfc)
  MATLAB Function/3(Ibatt_3) -> [curr_batt_command_3]
  From25/1 -> Sum1/2  "Batt current command 3"
  BATT/1 -> Bus Selector1/1
  Sum3/1 -> Ifc_conv/1
  [Vfc_conv] -> Vfc_conv/1
  Sum2/1 -> MATLAB Function1/1(current_comm)  "Batt current command"
  Bus Selector/1 -> [Vfc]  "<Vfc>"
  [Pload_real] -> PV - FC - control/13(Pout_real)
  [Ibatt] -> PV - FC - control/6(Ibatt_in)
  [Vpv] -> MATLAB Function/5(Vpv)
  [Vbus_real] -> MATLAB Function/9(Vdc)
  Discrete PI Controller7/1(Out) -> Sum3/2
  Bus Selector1/1 -> [Vbatt]  "<Voltage (V)>"
  Sum9/1 -> Sum8/1
  [Converter] -> batt converter mode/1
  MATLAB Function1/1(conv) -> [Converter]
  Constant/1 -> PV - FC - control/14(IO_pv_conv_value)
  [I_batt_charge] -> Ibatt_conv/1
  From30/1 -> Sum6/2, Sum7/2
  Discrete PI Controller1/1(Out) -> Sum9/1

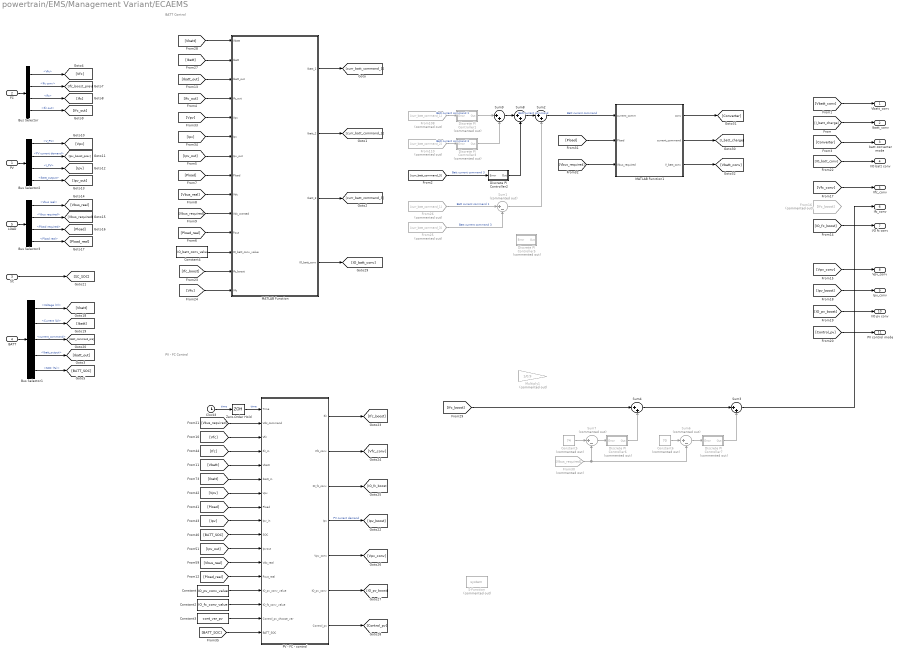
== system powertrain/EMS/Management Variant/ECAEMS ==
  note: PV - FC Control
  note: BATT Control
  PV : Inport
  FC : Inport  Port=2
  SC : Inport  Port=3
  BATT : Inport  Port=4
  LOAD : Inport  Port=5
  Bus Selector : BusSelector  OutputSignals=Vfc,Ifc conv,Ifc,Ifc out
  Bus Selector1 : BusSelector  OutputSignals=Voltage (V),Current (A),current_command,Ibatt_output,SOC (%)
  Bus Selector2 : BusSelector  OutputSignals=V_PV,PV current demand,I_PV,Ibatt_output
  Bus Selector3 : BusSelector  OutputSignals=Vbus real,Vbus required,Pload required,Pload real
  Clock3 : Clock
  Constant : Constant  Value=IO_pv_conv_value
  Constant2 : Constant  Value=IO_fc_conv_value
  Constant3 : Constant  Value=cont_var_pv
  Constant4 : Constant  Value=IO_batt_conv_value
  Constant5 : Constant  Commented=on  Value=74
  Constant6 : Constant  Commented=on  Value=70
  Discrete PI Controller1 : Subsystem  Commented=on  DialogController=POWERSYS.PowerSysDialog  mask(Discrete PI Controller){Kp=1, Ki=10, Par_Limits=[100 -100], Init=0, Ts=1e-4}
      mask prompts: Kp "Proportional gain (Kp):"; Ki "Integral gain (Ki):"; Par_Limits "Output limits: [ Upper   Lower ]"; Init "Output initial value:"; Ts "Sample time:"
      mask help: This block implements a discrete PI controller.
      mask init:
      | UpperLimit=Par_Limits(1);
      | LowerLimit=Par_Limits(2);
      | power_initmask();
      mask Help: This block is part of a subset of blocks in the Extras library that does not have documentation associated with it, other than the block mask description.
      mask Display: disp('PI');
  Discrete PI Controller2 : Subsystem  DialogController=POWERSYS.PowerSysDialog  mask(Discrete PI Controller){Kp=10, Ki=100, Par_Limits=[30 -4], Init=0, Ts=Ts}
      mask prompts: Kp "Proportional gain (Kp):"; Ki "Integral gain (Ki):"; Par_Limits "Output limits: [ Upper   Lower ]"; Init "Output initial value:"; Ts "Sample time:"
      mask help: This block implements a discrete PI controller.
      mask init:
      | UpperLimit=Par_Limits(1);
      | LowerLimit=Par_Limits(2);
      | power_initmask();
      mask Help: This block is part of a subset of blocks in the Extras library that does not have documentation associated with it, other than the block mask description.
      mask Display: disp('PI');
  Discrete PI Controller3 : Subsystem  Commented=on  DialogController=POWERSYS.PowerSysDialog  mask(Discrete PI Controller){Kp=10, Ki=1, Par_Limits=[100 -100], Init=0, Ts=1e-4}
      mask prompts: Kp "Proportional gain (Kp):"; Ki "Integral gain (Ki):"; Par_Limits "Output limits: [ Upper   Lower ]"; Init "Output initial value:"; Ts "Sample time:"
      mask help: This block implements a discrete PI controller.
      mask init:
      | UpperLimit=Par_Limits(1);
      | LowerLimit=Par_Limits(2);
      | power_initmask();
      mask Help: This block is part of a subset of blocks in the Extras library that does not have documentation associated with it, other than the block mask description.
      mask Display: disp('PI');
  Discrete PI Controller5 : Subsystem  Commented=on  DialogController=POWERSYS.PowerSysDialog  mask(Discrete PI Controller){Kp=10, Ki=10, Par_Limits=[50 -20], Init=0, Ts=1e-4}
      mask prompts: Kp "Proportional gain (Kp):"; Ki "Integral gain (Ki):"; Par_Limits "Output limits: [ Upper   Lower ]"; Init "Output initial value:"; Ts "Sample time:"
      mask help: This block implements a discrete PI controller.
      mask init:
      | UpperLimit=Par_Limits(1);
      | LowerLimit=Par_Limits(2);
      | power_initmask();
      mask Help: This block is part of a subset of blocks in the Extras library that does not have documentation associated with it, other than the block mask description.
      mask Display: disp('PI');
  Discrete PI Controller6 : Subsystem  Commented=on  DialogController=POWERSYS.PowerSysDialog  mask(Discrete PI Controller){Kp=10, Ki=10, Par_Limits=[40 0], Init=0, Ts=1e-4}
      mask prompts: Kp "Proportional gain (Kp):"; Ki "Integral gain (Ki):"; Par_Limits "Output limits: [ Upper   Lower ]"; Init "Output initial value:"; Ts "Sample time:"
      mask help: This block implements a discrete PI controller.
      mask init:
      | UpperLimit=Par_Limits(1);
      | LowerLimit=Par_Limits(2);
      | power_initmask();
      mask Help: This block is part of a subset of blocks in the Extras library that does not have documentation associated with it, other than the block mask description.
      mask Display: disp('PI');
  Discrete PI Controller7 : Subsystem  Commented=on  DialogController=POWERSYS.PowerSysDialog  mask(Discrete PI Controller){Kp=10, Ki=10, Par_Limits=[0 -40], Init=0, Ts=1e-4}
      mask prompts: Kp "Proportional gain (Kp):"; Ki "Integral gain (Ki):"; Par_Limits "Output limits: [ Upper   Lower ]"; Init "Output initial value:"; Ts "Sample time:"
      mask help: This block implements a discrete PI controller.
      mask init:
      | UpperLimit=Par_Limits(1);
      | LowerLimit=Par_Limits(2);
      | power_initmask();
      mask Help: This block is part of a subset of blocks in the Extras library that does not have documentation associated with it, other than the block mask description.
      mask Display: disp('PI');
  From108 : From  Commented=on  GotoTag=curr_batt_command_1
  From110 : From  Commented=on  GotoTag=curr_batt_command_2
  From16 : From  Commented=on  GotoTag=Ifc_boost
  From25 : From  Commented=on  GotoTag=curr_batt_command_3
  From26 : From  Commented=on  GotoTag=curr_batt_command_1
  From30 : From  Commented=on  GotoTag=Vbus_required
  MATLAB Function : MATLAB Function  TreatAsAtomicUnit=on
  MATLAB Function1 : MATLAB Function  TreatAsAtomicUnit=on
  Multiply1 : Gain  Commented=on  Gain=1/0.9
  PV - FC - control : MATLAB Function  TreatAsAtomicUnit=on
  S-Function : S-Function  Commented=on  SFunctionDeploymentMode=off  EnableBusSupport=off
  Sum1 : Sum  Commented=on  Inputs=|+-
  Sum{2..4,8..9} (5 alike) : Sum  Inputs=|++
  Sum6 : Sum  Commented=on  Inputs=|+-
  Sum7 : Sum  Commented=on  Inputs=|+-
  Zero-Order Hold : ZeroOrderHold  SampleTime=Ts
  Vbatt_conv : Outport
  Ibatt_conv : Outport  Port=2
  batt converter mode : Outport  Port=3
  I/O batt conv : Outport  Port=4
  Vfc_conv : Outport  Port=5
  Ifc_conv : Outport  Port=6
  I/O fc conv : Outport  Port=7
  Vpv_conv : Outport  Port=8
  Ipv_conv : Outport  Port=9
  I/O pv conv : Outport  Port=10
  PV control mode : Outport  Port=11
  wires:
  PV - FC - control/1(Ifc) -> [Ifc_boost]
  [Ipv_boost] -> Ipv_conv/1
  [Ifc_boost] -> MATLAB Function/13(Ifc_boost)
  [BATT_SOC] -> PV - FC - control/10(SOC)
  FC/1 -> Bus Selector/1
  Bus Selector2/2 -> [Ipv_boost_prev]  "<PV current demand>"
  Constant3/1 -> PV - FC - control/16(Control_pv_choose_var)
  Bus Selector3/4 -> [Pload_real]  "<Pload real>"
  Bus Selector1/5 -> [BATT_SOC]  "<SOC (%)>"
  [Ifc] -> PV - FC - control/4(Ifc_in)
  [Vbatt] -> PV - FC - control/5(Vbatt)
  MATLAB Function1/3(V_batt_conv) -> [Vbatt_conv]
  From26/1 -> Sum1/1  "Batt current command 1"
  PV - FC - control/2(Vfc_conv) -> [Vfc_conv]
  LOAD/1 -> Bus Selector3/1
  [BATT_SOC] -> PV - FC - control/17(BATT_SOC)
  Bus Selector3/3 -> [Pload]  "<Pload required>"
  [Ifc_boost] -> Sum4/1
  [Ipv_out] -> MATLAB Function/7(Ipv_out)
  PV/1 -> Bus Selector2/1
  [IO_batt_conv] -> I/O batt conv/1
  [Vpv_conv] -> Vpv_conv/1
  [Vbus_required] -> MATLAB Function1/3(Vbus_required)
  [Vbus_required] -> MATLAB Function/10(Vdc_wanted)
  Bus Selector/3 -> [Ifc]  "<Ifc>"
  From110/1 -> Discrete PI Controller3/1(Error)  "Batt current command 3"
  [Control_pv] -> PV control mode/1
  PV - FC - control/3(IO_fc_conv) -> [IO_fc_boost]
  PV - FC - control/4(Ipv) -> [Ipv_boost]  "PV current demand"
  [Pload] -> MATLAB Function/8(Pload)
  PV - FC - control/7(Control_pv) -> [Control_pv]
  [Vpv] -> PV - FC - control/7(Vpv)
  Zero-Order Hold/1 -> PV - FC - control/1(Time)  "time"
  MATLAB Function/4(IO_batt_conv) -> [IO_batt_conv]
  Clock3/1 -> Zero-Order Hold/1  "time"
  [Ipv] -> PV - FC - control/9(Ipv_in)
  Sum1/1 -> Sum2/2
  [Ipv_out] -> PV - FC - control/11(Ipvout)
  [Pload] -> MATLAB Function1/2(Pload)
  Constant5/1 -> Sum7/1
  Sum7/1 -> Discrete PI Controller6/1(Error)
  Sum3/1 -> Ifc_conv/1
  BATT/1 -> Bus Selector1/1
  Constant6/1 -> Sum6/1
  MATLAB Function/1(Ibatt_1) -> [curr_batt_command_1]
  Sum8/1 -> Sum2/1  "Batt current command"
  Sum2/1 -> MATLAB Function1/1(current_comm)  "Batt current command"
  [Vbus_real] -> PV - FC - control/12(Vdc_real)
  From25/1 -> Sum1/2  "Batt current command 3"
  [Ipv] -> MATLAB Function/6(Ipv)
  [IO_pv_boost] -> I/O pv conv/1
  Bus Selector2/3 -> [Ipv]  "<I_PV>"
  MATLAB Function/2(Ibatt_2) -> [curr_batt_command_2]
  Discrete PI Controller3/1(Out) -> Sum9/2
  [IO_fc_boost] -> I/O fc conv/1
  From108/1 -> Discrete PI Controller1/1(Error)  "Batt current command 1"
  [Ibatt] -> MATLAB Function/2(Ibatt)
  Sum6/1 -> Discrete PI Controller7/1(Error)
  Constant2/1 -> PV - FC - control/15(IO_fc_conv_value)
  PV - FC - control/6(IO_pv_conv) -> [IO_pv_boost]
  SC/1 -> [SC_SOC]
  Bus Selector1/4 -> [Ibatt_out]  "<Ibatt_output>"
  Bus Selector/4 -> [Ifc_out]  "<Ifc out>"
  PV - FC - control/5(Vpv_conv) -> [Vpv_conv]
  Bus Selector2/4 -> [Ipv_out]  "<Ibatt_output>"
  Bus Selector/2 -> [Ifc_boost_prev]  "<Ifc conv>"
  Bus Selector3/1 -> [Vbus_real]  "<Vbus real>"
  Bus Selector3/2 -> [Vbus_required]  "<Vbus required>"
  Bus Selector1/2 -> [Ibatt]  "<Current (A)>"
  Bus Selector2/1 -> [Vpv]  "<V_PV>"
  [Pload_real] -> MATLAB Function/11(Pout)
  Bus Selector1/3 -> [Ibatt_command_pre]  "<current_command>"
  Bus Selector/1 -> [Vfc]  "<Vfc>"
  Constant/1 -> PV - FC - control/14(IO_pv_conv_value)
  [Pload] -> PV - FC - control/8(Pload)
  Sum4/1 -> Sum3/1
  Sum9/1 -> Sum8/1
  [Vpv] -> MATLAB Function/5(Vpv)
  From30/1 -> Sum6/2, Sum7/2
  [Vbatt_conv] -> Vbatt_conv/1
  [Ibatt] -> PV - FC - control/6(Ibatt_in)
  Discrete PI Controller2/1(Out) -> Sum8/2
  MATLAB Function/3(Ibatt_3) -> [curr_batt_command_3]
  [Vfc] -> MATLAB Function/14(Vfc)
  Bus Selector1/1 -> [Vbatt]  "<Voltage (V)>"
  [Vfc_conv] -> Vfc_conv/1
  [I_batt_charge] -> Ibatt_conv/1
  Discrete PI Controller1/1(Out) -> Sum9/1
  Constant4/1 -> MATLAB Function/12(IO_batt_conv_value)
  [curr_batt_command_3] -> Discrete PI Controller2/1(Error)  "Batt current command 3"
  [Vfc] -> PV - FC - control/3(Vfc)
  [Pload_real] -> PV - FC - control/13(Pout_real)
  [Ifc_out] -> MATLAB Function/4(Ifc_out)
  [Vbus_required] -> PV - FC - control/2(Vdc_command)
  Discrete PI Controller6/1(Out) -> Sum4/2
  Discrete PI Controller7/1(Out) -> Sum3/2
  [Vbus_real] -> MATLAB Function/9(Vdc)
  [Vbatt] -> MATLAB Function/1(Vbatt)
  MATLAB Function1/2(current_command) -> [I_batt_charge]
  [Ibatt_out] -> MATLAB Function/3(Ibatt_out)
  [Converter] -> batt converter mode/1
  MATLAB Function1/1(conv) -> [Converter]
